simulink model "IEEE9_case"  (R2024b)
settings: Solver=FixedStepAuto  StartTime=0  StopTime=5  FixedStep=1e-7  RelTol=1e-3
values from neighbouring files (symbols this model uses):
  SG_D_1_D = 0.01056    [IEEE9_case_parameters.m]    (also in case1_parameters.m; case2_parameters.m; case3_parameters.m; case4_parameters.m)
  SG_D_1_EnableSaturation = 0    [IEEE9_case_parameters.m]    (also in case1_parameters.m; case2_parameters.m; case3_parameters.m; case4_parameters.m)
  SG_D_1_f0 = 60    [IEEE9_case_parameters.m]    (also in case1_parameters.m; case2_parameters.m; case3_parameters.m; case4_parameters.m)
  SG_D_1_H = 7.5    [IEEE9_case_parameters.m]    (also in case1_parameters.m; case2_parameters.m; case3_parameters.m; case4_parameters.m)
  SG_D_1_K_A = 20    [IEEE9_case_parameters.m]    (also in case1_parameters.m; case2_parameters.m; case3_parameters.m; case4_parameters.m)
  SG_D_1_K_E = 1.000000e+1    (= 10)    [IEEE9_case_parameters.m]    (also in case1_parameters.m; case2_parameters.m; case3_parameters.m; case4_parameters.m)
  SG_D_1_K_F = 2.363    [IEEE9_case_parameters.m]    (also in case1_parameters.m; case2_parameters.m; case3_parameters.m; case4_parameters.m)
  SG_D_1_K_s = 0.5    [IEEE9_case_parameters.m]    (also in case1_parameters.m = 5; case2_parameters.m = 5; case3_parameters.m = 5; case4_parameters.m = 5)
  SG_D_1_R_a = 0.001088    [IEEE9_case_parameters.m]    (also in case1_parameters.m; case2_parameters.m; case3_parameters.m; case4_parameters.m)
  SG_D_1_S_A = 1    [IEEE9_case_parameters.m]    (also in case1_parameters.m; case2_parameters.m; case3_parameters.m; case4_parameters.m)
  SG_D_1_S_B = 0.103    [IEEE9_case_parameters.m]    (also in case1_parameters.m; case2_parameters.m; case3_parameters.m; case4_parameters.m)
  SG_D_1_S_N = 10.659857    [IEEE9_case_parameters.m]    (also in case1_parameters.m; case2_parameters.m; case3_parameters.m; case4_parameters.m)
  SG_D_1_SpeedPara = 200    [IEEE9_case_parameters.m]    (also in case1_parameters.m; case2_parameters.m; case3_parameters.m; case4_parameters.m)
  SG_D_1_T_0 = 0.720173    [IEEE9_case_parameters.m]    (also in case1_parameters.m = 0.755522; case2_parameters.m = 0.808931; case3_parameters.m = 0.869402; case4_parameters.m = 0.729316)
  SG_D_1_T_1 = 0.3    [IEEE9_case_parameters.m]    (also in case1_parameters.m; case2_parameters.m; case3_parameters.m; case4_parameters.m)
  SG_D_1_T_2 = 0.05    [IEEE9_case_parameters.m]    (also in case1_parameters.m; case2_parameters.m; case3_parameters.m; case4_parameters.m)
  SG_D_1_T_3 = 0.02    [IEEE9_case_parameters.m]    (also in case1_parameters.m; case2_parameters.m; case3_parameters.m; case4_parameters.m)
  SG_D_1_T_4 = 0.005    [IEEE9_case_parameters.m]    (also in case1_parameters.m; case2_parameters.m; case3_parameters.m; case4_parameters.m)
  SG_D_1_T_A = 0.02    [IEEE9_case_parameters.m]    (also in case1_parameters.m; case2_parameters.m; case3_parameters.m; case4_parameters.m)
  SG_D_1_T_dd = 8.000000e+0    (= 8)    [IEEE9_case_parameters.m]    (also in case1_parameters.m; case2_parameters.m; case3_parameters.m; case4_parameters.m)
  SG_D_1_T_ddd = 0.04    [IEEE9_case_parameters.m]    (also in case1_parameters.m; case2_parameters.m; case3_parameters.m; case4_parameters.m)
  SG_D_1_T_E = 0.314    [IEEE9_case_parameters.m]    (also in case1_parameters.m; case2_parameters.m; case3_parameters.m; case4_parameters.m)
  SG_D_1_T_F = 0.35    [IEEE9_case_parameters.m]    (also in case1_parameters.m; case2_parameters.m; case3_parameters.m; case4_parameters.m)
  SG_D_1_T_qd = 0.8    [IEEE9_case_parameters.m]    (also in case1_parameters.m; case2_parameters.m; case3_parameters.m; case4_parameters.m)
  SG_D_1_T_qdd = 0.02    [IEEE9_case_parameters.m]    (also in case1_parameters.m; case2_parameters.m; case3_parameters.m; case4_parameters.m)
  SG_D_1_T_speed = 0.1    [IEEE9_case_parameters.m]    (also in case1_parameters.m = 200; case2_parameters.m = 200; case3_parameters.m = 200; case4_parameters.m = 200)
  SG_D_1_T_w = 0.5    [IEEE9_case_parameters.m]    (also in case1_parameters.m; case2_parameters.m; case3_parameters.m; case4_parameters.m)
  SG_D_1_V_ref = 1.990276    [IEEE9_case_parameters.m]    (also in case1_parameters.m = 2.042296; case2_parameters.m = 2.051388; case3_parameters.m = 2.089584; case4_parameters.m = 2.01845)
  SG_D_1_w_ref = 376.991118    [IEEE9_case_parameters.m]    (also in case1_parameters.m; case2_parameters.m; case3_parameters.m; case4_parameters.m)
  SG_D_1_wb = 6.000000e+1    (= 60)    [IEEE9_case_parameters.m]    (also in case1_parameters.m; case2_parameters.m; case3_parameters.m; case4_parameters.m)
  SG_D_1_x_d = 1.9    [IEEE9_case_parameters.m]    (also in case1_parameters.m; case2_parameters.m; case3_parameters.m; case4_parameters.m)
  SG_D_1_x_dd = 0.302    [IEEE9_case_parameters.m]    (also in case1_parameters.m; case2_parameters.m; case3_parameters.m; case4_parameters.m)
  SG_D_1_x_ddd = 0.204    [IEEE9_case_parameters.m]    (also in case1_parameters.m; case2_parameters.m; case3_parameters.m; case4_parameters.m)
  SG_D_1_x_l = 0.05    [IEEE9_case_parameters.m]    (also in case1_parameters.m; case2_parameters.m; case3_parameters.m; case4_parameters.m)
  SG_D_1_x_q = 1.3    [IEEE9_case_parameters.m]    (also in case1_parameters.m; case2_parameters.m; case3_parameters.m; case4_parameters.m)
  SG_D_1_x_qd = 0.5    [IEEE9_case_parameters.m]    (also in case1_parameters.m; case2_parameters.m; case3_parameters.m; case4_parameters.m)
  SG_D_1_x_qdd = 0.3    [IEEE9_case_parameters.m]    (also in case1_parameters.m; case2_parameters.m; case3_parameters.m; case4_parameters.m)
  SG_D_2_D = 0.02    [IEEE9_case_parameters.m]    (also in case1_parameters.m; case2_parameters.m; case3_parameters.m; case4_parameters.m)
  SG_D_2_EnableSaturation = 0    [IEEE9_case_parameters.m]    (also in case1_parameters.m; case2_parameters.m; case3_parameters.m; case4_parameters.m)
  SG_D_2_f0 = 60    [IEEE9_case_parameters.m]    (also in case1_parameters.m; case2_parameters.m; case3_parameters.m; case4_parameters.m)
  SG_D_2_H = 8.000000e+0    (= 8)    [IEEE9_case_parameters.m]    (also in case1_parameters.m; case2_parameters.m; case3_parameters.m; case4_parameters.m)
  SG_D_2_K_A = 20    [IEEE9_case_parameters.m]    (also in case1_parameters.m; case2_parameters.m; case3_parameters.m; case4_parameters.m)
  SG_D_2_K_E = 1.000000e+1    (= 10)    [IEEE9_case_parameters.m]    (also in case1_parameters.m; case2_parameters.m; case3_parameters.m; case4_parameters.m)
  SG_D_2_K_F = 2.363    [IEEE9_case_parameters.m]    (also in case1_parameters.m; case2_parameters.m; case3_parameters.m; case4_parameters.m)
  SG_D_2_K_s = 0.5    [IEEE9_case_parameters.m]    (also in case1_parameters.m = 4; case2_parameters.m = 4; case3_parameters.m = 4; case4_parameters.m = 4)
  SG_D_2_R_a = 0.001088    [IEEE9_case_parameters.m]    (also in case1_parameters.m; case2_parameters.m; case3_parameters.m; case4_parameters.m)
  SG_D_2_S_A = 1    [IEEE9_case_parameters.m]    (also in case1_parameters.m; case2_parameters.m; case3_parameters.m; case4_parameters.m)
  SG_D_2_S_B = 0.103    [IEEE9_case_parameters.m]    (also in case1_parameters.m; case2_parameters.m; case3_parameters.m; case4_parameters.m)
  SG_D_2_S_N = 10.659857    [IEEE9_case_parameters.m]    (also in case1_parameters.m; case2_parameters.m; case3_parameters.m; case4_parameters.m)
  SG_D_2_SpeedPara = 200    [IEEE9_case_parameters.m]    (also in case1_parameters.m; case2_parameters.m; case3_parameters.m; case4_parameters.m)
  SG_D_2_T_0 = 1.632913    [IEEE9_case_parameters.m]    (also in case1_parameters.m = 1.632925; case2_parameters.m = 1.632915; case3_parameters.m = 1.632914; case4_parameters.m = 1.632927)
  SG_D_2_T_1 = 0.2    [IEEE9_case_parameters.m]    (also in case1_parameters.m; case2_parameters.m; case3_parameters.m; case4_parameters.m)
  SG_D_2_T_2 = 0.05    [IEEE9_case_parameters.m]    (also in case1_parameters.m; case2_parameters.m; case3_parameters.m; case4_parameters.m)
  SG_D_2_T_3 = 0.02    [IEEE9_case_parameters.m]    (also in case1_parameters.m; case2_parameters.m; case3_parameters.m; case4_parameters.m)
  SG_D_2_T_4 = 0.005    [IEEE9_case_parameters.m]    (also in case1_parameters.m; case2_parameters.m; case3_parameters.m; case4_parameters.m)
  SG_D_2_T_A = 0.02    [IEEE9_case_parameters.m]    (also in case1_parameters.m; case2_parameters.m; case3_parameters.m; case4_parameters.m)
  SG_D_2_T_dd = 7.9    [IEEE9_case_parameters.m]    (also in case1_parameters.m; case2_parameters.m; case3_parameters.m; case4_parameters.m)
  SG_D_2_T_ddd = 0.04    [IEEE9_case_parameters.m]    (also in case1_parameters.m; case2_parameters.m; case3_parameters.m; case4_parameters.m)
  SG_D_2_T_E = 0.314    [IEEE9_case_parameters.m]    (also in case1_parameters.m; case2_parameters.m; case3_parameters.m; case4_parameters.m)
  SG_D_2_T_F = 0.35    [IEEE9_case_parameters.m]    (also in case1_parameters.m; case2_parameters.m; case3_parameters.m; case4_parameters.m)
  SG_D_2_T_qd = 0.8    [IEEE9_case_parameters.m]    (also in case1_parameters.m; case2_parameters.m; case3_parameters.m; case4_parameters.m)
  SG_D_2_T_qdd = 0.015    [IEEE9_case_parameters.m]    (also in case1_parameters.m; case2_parameters.m; case3_parameters.m; case4_parameters.m)
  SG_D_2_T_speed = 0.1    [IEEE9_case_parameters.m]    (also in case1_parameters.m = 150; case2_parameters.m = 150; case3_parameters.m = 150; case4_parameters.m = 150)
  SG_D_2_T_w = 0.35    [IEEE9_case_parameters.m]    (also in case1_parameters.m; case2_parameters.m; case3_parameters.m; case4_parameters.m)
  SG_D_2_V_ref = 2.58547    [IEEE9_case_parameters.m]    (also in case1_parameters.m = 2.597896; case2_parameters.m = 2.587136; case3_parameters.m = 2.586042; case4_parameters.m = 2.599679)
  SG_D_2_w_ref = 376.991118    [IEEE9_case_parameters.m]    (also in case1_parameters.m; case2_parameters.m; case3_parameters.m; case4_parameters.m)
  SG_D_2_wb = 6.000000e+1    (= 60)    [IEEE9_case_parameters.m]    (also in case1_parameters.m; case2_parameters.m; case3_parameters.m; case4_parameters.m)
  SG_D_2_x_d = 1.8    [IEEE9_case_parameters.m]    (also in case1_parameters.m; case2_parameters.m; case3_parameters.m; case4_parameters.m)
  SG_D_2_x_dd = 0.302    [IEEE9_case_parameters.m]    (also in case1_parameters.m; case2_parameters.m; case3_parameters.m; case4_parameters.m)
  SG_D_2_x_ddd = 0.204    [IEEE9_case_parameters.m]    (also in case1_parameters.m; case2_parameters.m; case3_parameters.m; case4_parameters.m)
  SG_D_2_x_l = 0.05    [IEEE9_case_parameters.m]    (also in case1_parameters.m; case2_parameters.m; case3_parameters.m; case4_parameters.m)
  SG_D_2_x_q = 1.25    [IEEE9_case_parameters.m]    (also in case1_parameters.m; case2_parameters.m; case3_parameters.m; case4_parameters.m)
  SG_D_2_x_qd = 0.5    [IEEE9_case_parameters.m]    (also in case1_parameters.m; case2_parameters.m; case3_parameters.m; case4_parameters.m)
  SG_D_2_x_qdd = 0.3    [IEEE9_case_parameters.m]    (also in case1_parameters.m; case2_parameters.m; case3_parameters.m; case4_parameters.m)
  SG_D_3_D = 0.02    [IEEE9_case_parameters.m]    (also in case1_parameters.m; case2_parameters.m; case3_parameters.m; case4_parameters.m)
  SG_D_3_EnableSaturation = 0    [IEEE9_case_parameters.m]    (also in case1_parameters.m; case2_parameters.m; case3_parameters.m; case4_parameters.m)
  SG_D_3_f0 = 60    [IEEE9_case_parameters.m]    (also in case1_parameters.m; case2_parameters.m; case3_parameters.m; case4_parameters.m)
  SG_D_3_H = 7.7    [IEEE9_case_parameters.m]    (also in case1_parameters.m; case2_parameters.m; case3_parameters.m; case4_parameters.m)
  SG_D_3_K_A = 20    [IEEE9_case_parameters.m]    (also in case1_parameters.m; case2_parameters.m; case3_parameters.m; case4_parameters.m)
  SG_D_3_K_E = 1.000000e+1    (= 10)    [IEEE9_case_parameters.m]    (also in case1_parameters.m; case2_parameters.m; case3_parameters.m; case4_parameters.m)
  SG_D_3_K_F = 2.363    [IEEE9_case_parameters.m]    (also in case1_parameters.m; case2_parameters.m; case3_parameters.m; case4_parameters.m)
  SG_D_3_K_s = 0.2    [IEEE9_case_parameters.m]    (also in case1_parameters.m = 2; case2_parameters.m = 2; case3_parameters.m = 2; case4_parameters.m = 2)
  SG_D_3_R_a = 0.001088    [IEEE9_case_parameters.m]    (also in case1_parameters.m; case2_parameters.m; case3_parameters.m; case4_parameters.m)
  SG_D_3_S_A = 1    [IEEE9_case_parameters.m]    (also in case1_parameters.m; case2_parameters.m; case3_parameters.m; case4_parameters.m)
  SG_D_3_S_B = 0.103    [IEEE9_case_parameters.m]    (also in case1_parameters.m; case2_parameters.m; case3_parameters.m; case4_parameters.m)
  SG_D_3_S_N = 10.659857    [IEEE9_case_parameters.m]    (also in case1_parameters.m; case2_parameters.m; case3_parameters.m; case4_parameters.m)
  SG_D_3_SpeedPara = 200    [IEEE9_case_parameters.m]    (also in case1_parameters.m; case2_parameters.m; case3_parameters.m; case4_parameters.m)
  SG_D_3_T_0 = 0.850788    [IEEE9_case_parameters.m]    (also in case1_parameters.m = 0.850786; case2_parameters.m = 0.850787; case3_parameters.m; case4_parameters.m = 0.850786)
  SG_D_3_T_1 = 0.2    [IEEE9_case_parameters.m]    (also in case1_parameters.m; case2_parameters.m; case3_parameters.m; case4_parameters.m)
  SG_D_3_T_2 = 0.05    [IEEE9_case_parameters.m]    (also in case1_parameters.m; case2_parameters.m; case3_parameters.m; case4_parameters.m)
  SG_D_3_T_3 = 0.02    [IEEE9_case_parameters.m]    (also in case1_parameters.m; case2_parameters.m; case3_parameters.m; case4_parameters.m)
  SG_D_3_T_4 = 0.005    [IEEE9_case_parameters.m]    (also in case1_parameters.m; case2_parameters.m; case3_parameters.m; case4_parameters.m)
  SG_D_3_T_A = 0.02    [IEEE9_case_parameters.m]    (also in case1_parameters.m; case2_parameters.m; case3_parameters.m; case4_parameters.m)
  SG_D_3_T_dd = 8.1    [IEEE9_case_parameters.m]    (also in case1_parameters.m; case2_parameters.m; case3_parameters.m; case4_parameters.m)
  SG_D_3_T_ddd = 0.04    [IEEE9_case_parameters.m]    (also in case1_parameters.m; case2_parameters.m; case3_parameters.m; case4_parameters.m)
  SG_D_3_T_E = 0.314    [IEEE9_case_parameters.m]    (also in case1_parameters.m; case2_parameters.m; case3_parameters.m; case4_parameters.m)
  SG_D_3_T_F = 0.35    [IEEE9_case_parameters.m]    (also in case1_parameters.m; case2_parameters.m; case3_parameters.m; case4_parameters.m)
  SG_D_3_T_qd = 0.8    [IEEE9_case_parameters.m]    (also in case1_parameters.m; case2_parameters.m; case3_parameters.m; case4_parameters.m)
  SG_D_3_T_qdd = 0.015    [IEEE9_case_parameters.m]    (also in case1_parameters.m; case2_parameters.m; case3_parameters.m; case4_parameters.m)
  SG_D_3_T_speed = 0.1    [IEEE9_case_parameters.m]    (also in case1_parameters.m = 180; case2_parameters.m = 180; case3_parameters.m = 180; case4_parameters.m = 180)
  SG_D_3_T_w = 0.4    [IEEE9_case_parameters.m]    (also in case1_parameters.m; case2_parameters.m; case3_parameters.m; case4_parameters.m)
  SG_D_3_V_ref = 1.892727    [IEEE9_case_parameters.m]    (also in case1_parameters.m = 1.906439; case2_parameters.m = 1.895535; case3_parameters.m = 1.892105; case4_parameters.m = 1.906598)
  SG_D_3_w_ref = 376.991118    [IEEE9_case_parameters.m]    (also in case1_parameters.m; case2_parameters.m; case3_parameters.m; case4_parameters.m)
  SG_D_3_wb = 6.000000e+1    (= 60)    [IEEE9_case_parameters.m]    (also in case1_parameters.m; case2_parameters.m; case3_parameters.m; case4_parameters.m)
  SG_D_3_x_d = 1.85    [IEEE9_case_parameters.m]    (also in case1_parameters.m; case2_parameters.m; case3_parameters.m; case4_parameters.m)
  SG_D_3_x_dd = 0.302    [IEEE9_case_parameters.m]    (also in case1_parameters.m; case2_parameters.m; case3_parameters.m; case4_parameters.m)
  SG_D_3_x_ddd = 0.204    [IEEE9_case_parameters.m]    (also in case1_parameters.m; case2_parameters.m; case3_parameters.m; case4_parameters.m)
  SG_D_3_x_l = 0.05    [IEEE9_case_parameters.m]    (also in case1_parameters.m; case2_parameters.m; case3_parameters.m; case4_parameters.m)
  SG_D_3_x_q = 1.2    [IEEE9_case_parameters.m]    (also in case1_parameters.m; case2_parameters.m; case3_parameters.m; case4_parameters.m)
  SG_D_3_x_qd = 0.5    [IEEE9_case_parameters.m]    (also in case1_parameters.m; case2_parameters.m; case3_parameters.m; case4_parameters.m)
  SG_D_3_x_qdd = 0.3    [IEEE9_case_parameters.m]    (also in case1_parameters.m; case2_parameters.m; case3_parameters.m; case4_parameters.m)
(part 10 of 12)

== system IEEE9_case/SG_D_3/d_R_f_SG_D_3_block ==
  note: d_R_f_SG_D_3 in IEEE9_case
      | $-\frac{R_{f,\mathrm{SG},D,3}-\frac{E_{\mathrm{fd},\mathrm{SG},D,3}\,K_{F}}{T_{F}}}{T_{F}}$
      | Automatically generated on 2025-11-01 08:50:13 .
  State_E_fd_SG_D_3_ddbea : Inport
  State_R_f_SG_D_3_c9e06 : Inport  Port=2
  Constant_K_F_22646 : Constant  Value=K_F
  Constant_T_F_0a0d1 : Constant  Value=T_F
  Constant_T_F_8804f : Constant  Value=T_F
  Divide_a64c1 : Product  Inputs=*/
  Divide_bf12f : Product  Inputs=*/
  Product_f7b73 : Product
  Subtract_0003f : Sum  Inputs=+-
  Blockout_d_R_f_SG_D_3_4784a : Outport
  wires:
  State_E_fd_SG_D_3_ddbea/1 -> Product_f7b73/1
  Constant_T_F_8804f/1 -> Divide_bf12f/2
  Constant_K_F_22646/1 -> Product_f7b73/2
  Product_f7b73/1 -> Divide_bf12f/1
  Divide_bf12f/1 -> Subtract_0003f/1
  State_R_f_SG_D_3_c9e06/1 -> Subtract_0003f/2
  Subtract_0003f/1 -> Divide_a64c1/1
  Constant_T_F_0a0d1/1 -> Divide_a64c1/2
  Divide_a64c1/1 -> Blockout_d_R_f_SG_D_3_4784a/1

== system IEEE9_case/SG_D_3/d_T_m_SG_D_3_block ==
  note: d_T_m_SG_D_3 in IEEE9_case
      | $-\frac{T_{m,\mathrm{SG},D,3}-T_{0}+\frac{\mathrm{SpeedPara}\,\left(w_{\mathrm{SG},D,3}-w_{\mathrm{ref}}\right)}{2\,f_{0}\,\pi }}{T_{\mathrm{speed}}}$
      | Automatically generated on 2025-11-01 08:50:04 .
  State_w_SG_D_3_50cf4 : Inport
  State_T_m_SG_D_3_a1980 : Inport  Port=2
  Add_41ff0 : Sum
  Add_ea0f0 : Sum
  Constant_-1_92da2 : Constant  Value=-1
  Constant_2.0_2378e : Constant  Value=2.0
  Constant_SpeedPara_095da : Constant  Value=SpeedPara
  Constant_T_0_75c83 : Constant  Value=T_0
  Constant_T_speed_09506 : Constant  Value=T_speed
  Constant_f0_b89eb : Constant  Value=f0
  Constant_pi_24d1e : Constant  Value=pi
  Constant_w_ref_fa68f : Constant  Value=w_ref
  Divide_5e003 : Product  Inputs=*/
  Divide_e250a : Product  Inputs=*/
  Product_43f4e : Product
  Product_b2d5f : Product
  Product_c70c6 : Product
  Product_f87e7 : Product
  Subtract_c06a0 : Sum  Inputs=+-
  Blockout_d_T_m_SG_D_3_5f1a1 : Outport
  wires:
  Constant_SpeedPara_095da/1 -> Product_f87e7/1
  Constant_-1_92da2/1 -> Product_b2d5f/1
  Constant_w_ref_fa68f/1 -> Add_ea0f0/2
  State_w_SG_D_3_50cf4/1 -> Product_b2d5f/2
  Constant_2.0_2378e/1 -> Product_c70c6/1
  Product_b2d5f/1 -> Add_ea0f0/1
  Constant_pi_24d1e/1 -> Product_c70c6/2
  Add_ea0f0/1 -> Product_f87e7/2
  Product_c70c6/1 -> Product_43f4e/1
  Constant_f0_b89eb/1 -> Product_43f4e/2
  Product_f87e7/1 -> Divide_e250a/1
  Product_43f4e/1 -> Divide_e250a/2
  Divide_e250a/1 -> Add_41ff0/1
  Constant_T_0_75c83/1 -> Add_41ff0/2
  Add_41ff0/1 -> Subtract_c06a0/1
  State_T_m_SG_D_3_a1980/1 -> Subtract_c06a0/2
  Subtract_c06a0/1 -> Divide_5e003/1
  Constant_T_speed_09506/1 -> Divide_5e003/2
  Divide_5e003/1 -> Blockout_d_T_m_SG_D_3_5f1a1/1

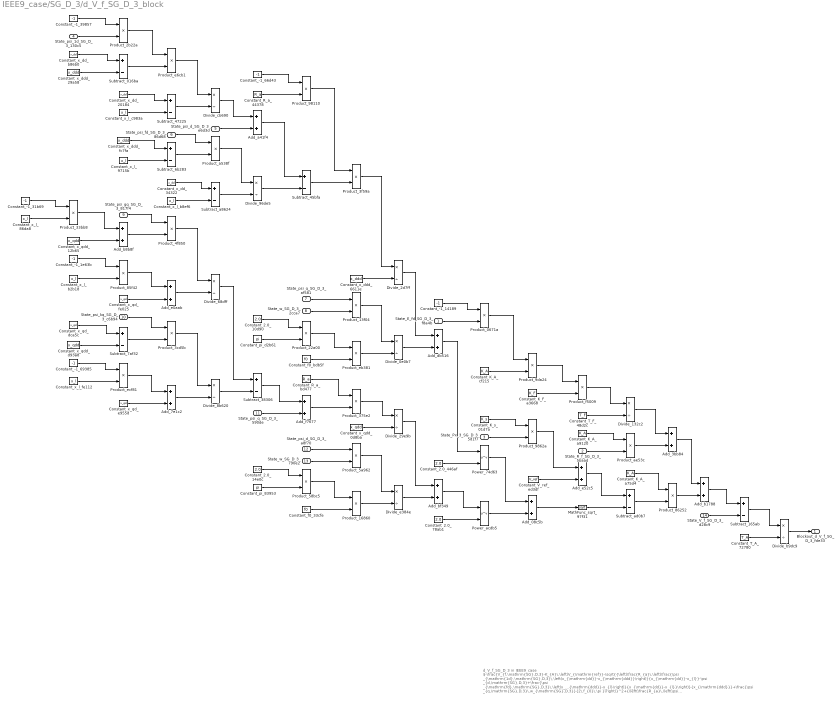
== system IEEE9_case/SG_D_3/d_V_f_SG_D_3_block ==
  note: d_V_f_SG_D_3 in IEEE9_case
      | $-\frac{V_{f,\mathrm{SG},D,3}-K_{A}\,\left(V_{\mathrm{ref}}-\sqrt{{\left(\frac{R_{a}\,\left(\frac{\psi _{\mathrm{1d},\mathrm{SG},D,3}\,\left(x_{\mathrm{dd}}-x_{\mathrm{ddd}}\right)}{x_{\mathrm{dd}}-x_{l}}-\psi _{d,\mathrm{SG},D,3}+\frac{\psi _{\mathrm{fd},\mathrm{SG},D,3}\,\left(x_{\mathrm{ddd}}-x_{l}\right)}{x_{\mathrm{dd}}-x_{l}}\right)}{x_{\mathrm{ddd}}}+\frac{\psi _{q,\mathrm{SG},D,3}\,w_{\mathrm{SG},D,3}}{2\,f_{0}\,\pi }\right)}^2+{\left(\frac{R_{a}\,\left(\psi _{q,\mathrm{SG},D,3}+\frac{\psi _{\mathrm{gq},\mathrm{SG},D,3}\,\left(x_{l}-x_{\mathrm{qdd}}\right)}{x_{l}-x_{\mathrm{qd}}}+\frac{\psi _{\mathrm{kq},\mathrm{SG},D,3}\,\left(x_{\mathrm{qd}}-x_{\mathrm{qdd}}\right)}{x_{l}-x_{\mathrm{qd}}}\right)}{x_{\mathrm{qdd}}}+\frac{\psi _{d,\mathrm{SG},D,3}\,w_{\mathrm{SG},D,3}}{2\,f_{0}\,\pi }\right)}^2}+K_{s}\,\mathrm{Px}_{3,\mathrm{SG},D,3}\right)-K_{A}\,R_{f,\mathrm{SG},D,3}+\frac{E_{\mathrm{fd},\mathrm{SG},D,3}\,K_{A}\,K_{F}}{T_{F}}}{T_{A}}$
      | Automatically generated on 2025-11-01 08:50:11 .
  State_E_fd_SG_D_3_f8a4b : Inport
  State_R_f_SG_D_3_5baad : Inport  Port=2
  State_Px_3_SG_D_3_5d1f7 : Inport  Port=3
  State_psi_1d_SG_D_3_130c5 : Inport  Port=4
  State_psi_d_SG_D_3_e6d3d : Inport  Port=5
  State_psi_fd_SG_D_3_86d68 : Inport  Port=6
  State_psi_q_SG_D_3_af581 : Inport  Port=7
  State_w_SG_D_3_2cca7 : Inport  Port=8
  State_psi_gq_SG_D_3_817f4 : Inport  Port=9
  State_psi_kq_SG_D_3_c6b94 : Inport  Port=10
  State_psi_q_SG_D_3_590de : Inport  Port=11
  State_psi_d_SG_D_3_a8f70 : Inport  Port=12
  State_w_SG_D_3_790e2 : Inport  Port=13
  State_V_f_SG_D_3_d28c9 : Inport  Port=14
  Add_08c5b : Sum
  Add_3bb84 : Sum
  Add_7e1c2 : Sum
  Add_a41f4 : Sum
  Add_b1788 : Sum
  Add_b8b8f : Sum
  Add_bf349 : Sum
  Add_db516 : Sum
  Add_e0aab : Sum
  Add_e52c5 : Sum
  Add_f7677 : Sum
  Constant_-1_14189 : Constant  Value=-1
  Constant_-1_1e63b : Constant  Value=-1
  Constant_-1_31b69 : Constant  Value=-1
  Constant_-1_39857 : Constant  Value=-1
  Constant_-1_66d43 : Constant  Value=-1
  Constant_-1_69385 : Constant  Value=-1
  Constant_2.0_10d90 : Constant  Value=2.0
  Constant_2.0_14e0c : Constant  Value=2.0
  Constant_2.0_446af : Constant  Value=2.0
  Constant_2.0_78ab1 : Constant  Value=2.0
  Constant_K_A_a75d4 : Constant  Value=K_A
  Constant_K_A_a9120 : Constant  Value=K_A
  Constant_K_A_cf215 : Constant  Value=K_A
  Constant_K_F_a3668 : Constant  Value=K_F
  Constant_K_s_01d7a : Constant  Value=K_s
  Constant_R_a_44378 : Constant  Value=R_a
  Constant_R_a_bd477 : Constant  Value=R_a
  Constant_T_A_72780 : Constant  Value=T_A
  Constant_T_F_48d2c : Constant  Value=T_F
  Constant_V_ref_ed3df : Constant  Value=V_ref
  Constant_f0_33cfe : Constant  Value=f0
  Constant_f0_bdb5f : Constant  Value=f0
  Constant_pi_83953 : Constant  Value=pi
  Constant_pi_d2b61 : Constant  Value=pi
  Constant_x_dd_20184 : Constant  Value=x_dd
  Constant_x_dd_34322 : Constant  Value=x_dd
  Constant_x_dd_b86b0 : Constant  Value=x_dd
  Constant_x_ddd_29a58 : Constant  Value=x_ddd
  Constant_x_ddd_6611e : Constant  Value=x_ddd
  Constant_x_ddd_fc7fa : Constant  Value=x_ddd
  Constant_x_l_86da8 : Constant  Value=x_l
  Constant_x_l_9715b : Constant  Value=x_l
  Constant_x_l_b2b18 : Constant  Value=x_l
  Constant_x_l_b8ef6 : Constant  Value=x_l
  Constant_x_l_c983a : Constant  Value=x_l
  Constant_x_l_fe112 : Constant  Value=x_l
  Constant_x_qd_dca5c : Constant  Value=x_qd
  Constant_x_qd_e955d : Constant  Value=x_qd
  Constant_x_qd_fe025 : Constant  Value=x_qd
  Constant_x_qdd_0d8ba : Constant  Value=x_qdd
  Constant_x_qdd_12b65 : Constant  Value=x_qdd
  Constant_x_qdd_d93a8 : Constant  Value=x_qdd
  Divide_0e0b7 : Product  Inputs=*/
  Divide_132c2 : Product  Inputs=*/
  Divide_29e9b : Product  Inputs=*/
  Divide_2d7ff : Product  Inputs=*/
  Divide_68dff : Product  Inputs=*/
  Divide_8b620 : Product  Inputs=*/
  Divide_96de5 : Product  Inputs=*/
  Divide_b9dc9 : Product  Inputs=*/
  Divide_cb690 : Product  Inputs=*/
  Divide_e384e : Product  Inputs=*/
  MathFunc_sqrt_97f31 : Sqrt
  Power_74d63 : Math  Operator=pow
  Power_acdb5 : Math  Operator=pow
  Product_0671a : Product
  Product_13f04 : Product
  Product_16860 : Product
  Product_22a00 : Product
  Product_2b22a : Product
  Product_33bb8 : Product
  Product_375e2 : Product
  Product_3cd5b : Product
  Product_3f59a : Product
  Product_4f850 : Product
  Product_58bc5 : Product
  Product_5a962 : Product
  Product_85f42 : Product
  Product_86252 : Product
  Product_98110 : Product
  Product_9862a : Product
  Product_9da24 : Product
  Product_a538f : Product
  Product_ae53c : Product
  Product_e6cb1 : Product
  Product_eb381 : Product
  Product_ecf81 : Product
  Product_f5009 : Product
  Subtract_016ba : Sum  Inputs=+-
  Subtract_165ab : Sum  Inputs=+-
  Subtract_38306 : Sum  Inputs=+-
  Subtract_45bfa : Sum  Inputs=+-
  Subtract_47225 : Sum  Inputs=+-
  Subtract_6b283 : Sum  Inputs=+-
  Subtract_7af32 : Sum  Inputs=+-
  Subtract_a8624 : Sum  Inputs=+-
  Subtract_ad0b7 : Sum  Inputs=+-
  Blockout_d_V_f_SG_D_3_fde33 : Outport
  wires:
  Constant_K_A_a9120/1 -> Product_ae53c/1
  Constant_-1_31b69/1 -> Product_33bb8/1
  Subtract_6b283/1 -> Product_a538f/2
  Constant_x_l_86da8/1 -> Product_33bb8/2
  Divide_e384e/1 -> Add_bf349/2
  Constant_-1_39857/1 -> Product_2b22a/1
  State_psi_1d_SG_D_3_130c5/1 -> Product_2b22a/2
  Constant_x_dd_b86b0/1 -> Subtract_016ba/1
  Divide_96de5/1 -> Subtract_45bfa/2
  Product_33bb8/1 -> Add_b8b8f/1
  Constant_x_qdd_12b65/1 -> Add_b8b8f/2
  Constant_x_ddd_29a58/1 -> Subtract_016ba/2
  Constant_2.0_78ab1/1 -> Power_acdb5/2
  Constant_-1_1e63b/1 -> Product_85f42/1
  Divide_68dff/1 -> Subtract_38306/1
  Subtract_47225/1 -> Divide_cb690/2
  Constant_x_l_b2b18/1 -> Product_85f42/2
  Constant_x_qd_dca5c/1 -> Subtract_7af32/1
  State_w_SG_D_3_2cca7/1 -> Product_13f04/2
  Constant_x_qdd_d93a8/1 -> Subtract_7af32/2
  Constant_2.0_10d90/1 -> Product_22a00/1
  Constant_-1_69385/1 -> Product_ecf81/1
  Constant_pi_d2b61/1 -> Product_22a00/2
  Add_a41f4/1 -> Subtract_45bfa/1
  Constant_x_l_fe112/1 -> Product_ecf81/2
  Product_2b22a/1 -> Product_e6cb1/1
  Subtract_016ba/1 -> Product_e6cb1/2
  Constant_2.0_14e0c/1 -> Product_58bc5/1
  Constant_x_dd_20184/1 -> Subtract_47225/1
  Constant_pi_83953/1 -> Product_58bc5/2
  Constant_x_l_c983a/1 -> Subtract_47225/2
  Constant_x_ddd_fc7fa/1 -> Subtract_6b283/1
  Constant_x_l_9715b/1 -> Subtract_6b283/2
  State_psi_gq_SG_D_3_817f4/1 -> Product_4f850/1
  Constant_x_l_b8ef6/1 -> Subtract_a8624/2
  Add_b8b8f/1 -> Product_4f850/2
  Product_85f42/1 -> Add_e0aab/1
  Product_4f850/1 -> Divide_68dff/1
  Constant_x_qd_fe025/1 -> Add_e0aab/2
  State_psi_kq_SG_D_3_c6b94/1 -> Product_3cd5b/1
  State_psi_q_SG_D_3_af581/1 -> Product_13f04/1
  Add_db516/1 -> Power_74d63/1
  Subtract_7af32/1 -> Product_3cd5b/2
  Constant_f0_bdb5f/1 -> Product_eb381/2
  Product_22a00/1 -> Product_eb381/1
  Constant_x_qd_e955d/1 -> Add_7e1c2/2
  Product_ecf81/1 -> Add_7e1c2/1
  Product_e6cb1/1 -> Divide_cb690/1
  State_psi_fd_SG_D_3_86d68/1 -> Product_a538f/1
  Constant_x_dd_34322/1 -> Subtract_a8624/1
  Add_e0aab/1 -> Divide_68dff/2
  Add_08c5b/1 -> MathFunc_sqrt_97f31/1
  Product_3cd5b/1 -> Divide_8b620/1
  Add_7e1c2/1 -> Divide_8b620/2
  Product_98110/1 -> Product_3f59a/1
  Divide_cb690/1 -> Add_a41f4/1
  Add_e52c5/1 -> Subtract_ad0b7/1
  State_psi_d_SG_D_3_e6d3d/1 -> Add_a41f4/2
  Product_a538f/1 -> Divide_96de5/1
  Subtract_a8624/1 -> Divide_96de5/2
  MathFunc_sqrt_97f31/1 -> Subtract_ad0b7/2
  Divide_8b620/1 -> Subtract_38306/2
  Constant_-1_66d43/1 -> Product_98110/1
  Constant_R_a_44378/1 -> Product_98110/2
  Subtract_38306/1 -> Add_f7677/1
  State_psi_q_SG_D_3_590de/1 -> Add_f7677/2
  Subtract_45bfa/1 -> Product_3f59a/2
  Constant_R_a_bd477/1 -> Product_375e2/1
  Add_f7677/1 -> Product_375e2/2
  State_psi_d_SG_D_3_a8f70/1 -> Product_5a962/1
  State_w_SG_D_3_790e2/1 -> Product_5a962/2
  Product_58bc5/1 -> Product_16860/1
  Constant_f0_33cfe/1 -> Product_16860/2
  Product_3f59a/1 -> Divide_2d7ff/1
  Constant_x_ddd_6611e/1 -> Divide_2d7ff/2
  Product_13f04/1 -> Divide_0e0b7/1
  Product_eb381/1 -> Divide_0e0b7/2
  Product_375e2/1 -> Divide_29e9b/1
  Constant_x_qdd_0d8ba/1 -> Divide_29e9b/2
  Product_5a962/1 -> Divide_e384e/1
  Product_16860/1 -> Divide_e384e/2
  Divide_2d7ff/1 -> Add_db516/1
  Divide_0e0b7/1 -> Add_db516/2
  Divide_29e9b/1 -> Add_bf349/1
  Constant_-1_14189/1 -> Product_0671a/1
  State_E_fd_SG_D_3_f8a4b/1 -> Product_0671a/2
  Constant_2.0_446af/1 -> Power_74d63/2
  Add_bf349/1 -> Power_acdb5/1
  Product_0671a/1 -> Product_9da24/1
  Constant_K_A_cf215/1 -> Product_9da24/2
  Constant_K_s_01d7a/1 -> Product_9862a/1
  State_Px_3_SG_D_3_5d1f7/1 -> Product_9862a/2
  Power_74d63/1 -> Add_08c5b/1
  Power_acdb5/1 -> Add_08c5b/2
  Product_9da24/1 -> Product_f5009/1
  Constant_K_F_a3668/1 -> Product_f5009/2
  Product_9862a/1 -> Add_e52c5/1
  Constant_V_ref_ed3df/1 -> Add_e52c5/2
  Product_f5009/1 -> Divide_132c2/1
  Constant_T_F_48d2c/1 -> Divide_132c2/2
  Add_b1788/1 -> Subtract_165ab/1
  State_R_f_SG_D_3_5baad/1 -> Product_ae53c/2
  Divide_132c2/1 -> Add_3bb84/1
  Product_ae53c/1 -> Add_3bb84/2
  Constant_K_A_a75d4/1 -> Product_86252/1
  Subtract_ad0b7/1 -> Product_86252/2
  Add_3bb84/1 -> Add_b1788/1
  Product_86252/1 -> Add_b1788/2
  State_V_f_SG_D_3_d28c9/1 -> Subtract_165ab/2
  Subtract_165ab/1 -> Divide_b9dc9/1
  Constant_T_A_72780/1 -> Divide_b9dc9/2
  Divide_b9dc9/1 -> Blockout_d_V_f_SG_D_3_fde33/1

== system IEEE9_case/SG_D_3/d_psi_1d_SG_D_3_block ==
  note: d_psi_1d_SG_D_3 in IEEE9_case
      | $-\frac{\psi _{\mathrm{1d},\mathrm{SG},D,3}-\psi _{\mathrm{fd},\mathrm{SG},D,3}+\frac{\left(x_{\mathrm{dd}}-x_{l}\right)\,\left(\frac{\psi _{\mathrm{1d},\mathrm{SG},D,3}\,\left(x_{\mathrm{dd}}-x_{\mathrm{ddd}}\right)}{x_{\mathrm{dd}}-x_{l}}-\psi _{d,\mathrm{SG},D,3}+\frac{\psi _{\mathrm{fd},\mathrm{SG},D,3}\,\left(x_{\mathrm{ddd}}-x_{l}\right)}{x_{\mathrm{dd}}-x_{l}}\right)}{x_{\mathrm{ddd}}}}{T_{\mathrm{ddd}}}$
      | Automatically generated on 2025-11-01 08:49:48 .
  State_psi_1d_SG_D_3_dcaf3 : Inport
  State_psi_fd_SG_D_3_cacc3 : Inport  Port=2
  State_psi_1d_SG_D_3_98130 : Inport  Port=3
  State_psi_d_SG_D_3_fbd14 : Inport  Port=4
  State_psi_fd_SG_D_3_9f125 : Inport  Port=5
  Add_15da8 : Sum
  Add_83c0c : Sum
  Add_a7352 : Sum
  Constant_-1_18e36 : Constant  Value=-1
  Constant_-1_dc142 : Constant  Value=-1
  Constant_T_ddd_806da : Constant  Value=T_ddd
  Constant_x_dd_4b99c : Constant  Value=x_dd
  Constant_x_dd_76a92 : Constant  Value=x_dd
  Constant_x_dd_af030 : Constant  Value=x_dd
  Constant_x_dd_f0d56 : Constant  Value=x_dd
  Constant_x_ddd_4ece0 : Constant  Value=x_ddd
  Constant_x_ddd_688f3 : Constant  Value=x_ddd
  Constant_x_ddd_b84f1 : Constant  Value=x_ddd
  Constant_x_l_8316f : Constant  Value=x_l
  Constant_x_l_95cb8 : Constant  Value=x_l
  Constant_x_l_b4d52 : Constant  Value=x_l
  Constant_x_l_eaaef : Constant  Value=x_l
  Divide_065c3 : Product  Inputs=*/
  Divide_14861 : Product  Inputs=*/
  Divide_3c16f : Product  Inputs=*/
  Divide_4ed99 : Product  Inputs=*/
  Product_14a64 : Product
  Product_74950 : Product
  Product_afc25 : Product
  Product_b95af : Product
  Product_d3848 : Product
  Subtract_0f08b : Sum  Inputs=+-
  Subtract_361bd : Sum  Inputs=+-
  Subtract_4fe76 : Sum  Inputs=+-
  Subtract_70533 : Sum  Inputs=+-
  Subtract_7fade : Sum  Inputs=+-
  Subtract_922fb : Sum  Inputs=+-
  Blockout_d_psi_1d_SG_D_3_549d8 : Outport
  wires:
  Divide_14861/1 -> Add_15da8/1
  Subtract_361bd/1 -> Product_afc25/2
  Constant_-1_dc142/1 -> Product_74950/1
  Constant_x_dd_f0d56/1 -> Subtract_4fe76/1
  State_psi_1d_SG_D_3_98130/1 -> Product_74950/2
  Product_74950/1 -> Product_afc25/1
  Constant_x_dd_76a92/1 -> Subtract_361bd/1
  Constant_x_ddd_688f3/1 -> Subtract_361bd/2
  Constant_x_l_95cb8/1 -> Subtract_4fe76/2
  Constant_x_ddd_b84f1/1 -> Subtract_70533/1
  Divide_3c16f/1 -> Blockout_d_psi_1d_SG_D_3_549d8/1
  Constant_x_l_b4d52/1 -> Subtract_70533/2
  Product_afc25/1 -> Divide_14861/1
  Subtract_4fe76/1 -> Divide_14861/2
  State_psi_fd_SG_D_3_9f125/1 -> Product_14a64/1
  Subtract_70533/1 -> Product_14a64/2
  Constant_x_dd_af030/1 -> Subtract_0f08b/1
  Constant_x_l_eaaef/1 -> Subtract_0f08b/2
  State_psi_d_SG_D_3_fbd14/1 -> Add_15da8/2
  Product_14a64/1 -> Divide_065c3/1
  Subtract_0f08b/1 -> Divide_065c3/2
  Constant_x_dd_4b99c/1 -> Subtract_922fb/1
  Constant_x_l_8316f/1 -> Subtract_922fb/2
  Add_15da8/1 -> Subtract_7fade/1
  Divide_065c3/1 -> Subtract_7fade/2
  Constant_-1_18e36/1 -> Product_d3848/1
  State_psi_1d_SG_D_3_dcaf3/1 -> Product_d3848/2
  State_psi_fd_SG_D_3_cacc3/1 -> Add_83c0c/2
  Subtract_922fb/1 -> Product_b95af/1
  Subtract_7fade/1 -> Product_b95af/2
  Product_d3848/1 -> Add_83c0c/1
  Product_b95af/1 -> Divide_4ed99/1
  Constant_x_ddd_4ece0/1 -> Divide_4ed99/2
  Add_83c0c/1 -> Add_a7352/1
  Divide_4ed99/1 -> Add_a7352/2
  Add_a7352/1 -> Divide_3c16f/1
  Constant_T_ddd_806da/1 -> Divide_3c16f/2

== system IEEE9_case/SG_D_3/d_psi_d_SG_D_3_block ==
  note: d_psi_d_SG_D_3 in IEEE9_case
      | $2\,\pi \,f_{0}\,\left(v_{d,\mathrm{SG},D,3}\,\sin\left(\theta _{\mathrm{SG},D,3}\right)-v_{q,\mathrm{SG},D,3}\,\cos\left(\theta _{\mathrm{SG},D,3}\right)+\frac{R_{a}\,\left(\frac{\psi _{\mathrm{1d},\mathrm{SG},D,3}\,\left(x_{\mathrm{dd}}-x_{\mathrm{ddd}}\right)}{x_{\mathrm{dd}}-x_{l}}-\psi _{d,\mathrm{SG},D,3}+\frac{\psi _{\mathrm{fd},\mathrm{SG},D,3}\,\left(x_{\mathrm{ddd}}-x_{l}\right)}{x_{\mathrm{dd}}-x_{l}}\right)}{x_{\mathrm{ddd}}}+\frac{\psi _{q,\mathrm{SG},D,3}\,w_{\mathrm{SG},D,3}}{2\,f_{0}\,\pi }\right)$
      | Automatically generated on 2025-11-01 08:49:39 .
  State_psi_1d_SG_D_3_ec6d7 : Inport
  State_psi_d_SG_D_3_cd386 : Inport  Port=2
  State_psi_fd_SG_D_3_f7fa4 : Inport  Port=3
  Input_v_d_SG_D_3_c1082 : Inport  Port=4
  State_theta_SG_D_3_79acd : Inport  Port=5
  Input_v_q_SG_D_3_d2650 : Inport  Port=6
  State_theta_SG_D_3_d0ec2 : Inport  Port=7
  State_psi_q_SG_D_3_63db3 : Inport  Port=8
  State_w_SG_D_3_c8b72 : Inport  Port=9
  Add_7d94c : Sum
  Add_c23eb : Sum
  Constant_-1_b66cc : Constant  Value=-1
  Constant_-2.0_d9ac7 : Constant  Value=-2.0
  Constant_2.0_7e810 : Constant  Value=2.0
  Constant_R_a_5fc7e : Constant  Value=R_a
  Constant_f0_5bc15 : Constant  Value=f0
  Constant_f0_8268e : Constant  Value=f0
  Constant_pi_02ee2 : Constant  Value=pi
  Constant_pi_d37fe : Constant  Value=pi
  Constant_x_dd_0ce51 : Constant  Value=x_dd
  Constant_x_dd_5686e : Constant  Value=x_dd
  Constant_x_dd_6e989 : Constant  Value=x_dd
  Constant_x_ddd_32dbf : Constant  Value=x_ddd
  Constant_x_ddd_6e6b5 : Constant  Value=x_ddd
  Constant_x_ddd_9b171 : Constant  Value=x_ddd
  Constant_x_l_1451d : Constant  Value=x_l
  Constant_x_l_c1c50 : Constant  Value=x_l
  Constant_x_l_e75f6 : Constant  Value=x_l
  Divide_30391 : Product  Inputs=*/
  Divide_bb8a0 : Product  Inputs=*/
  Divide_bebb2 : Product  Inputs=*/
  Divide_e0f9d : Product  Inputs=*/
  MathFunc_cos_fdc9f : Trigonometry  Operator=cos
  MathFunc_sin_20479 : Trigonometry
  Product_0c9b7 : Product
  Product_1403c : Product
  Product_1465a : Product
  Product_31711 : Product
  Product_485fb : Product
  Product_7d538 : Product
  Product_7f1be : Product
  Product_87be9 : Product
  Product_8f97a : Product
  Product_a0011 : Product
  Product_f637c : Product
  Product_f7ca5 : Product
  Subtract_09f13 : Sum  Inputs=+-
  Subtract_21e04 : Sum  Inputs=+-
  Subtract_30b02 : Sum  Inputs=+-
  Subtract_a3228 : Sum  Inputs=+-
  Subtract_b7ec2 : Sum  Inputs=+-
  Subtract_fc50a : Sum  Inputs=+-
  Subtract_ffcf7 : Sum  Inputs=+-
  Blockout_d_psi_d_SG_D_3_12622 : Outport
  wires:
  Constant_-1_b66cc/1 -> Product_0c9b7/1
  Constant_2.0_7e810/1 -> Product_87be9/1
  Constant_x_dd_5686e/1 -> Subtract_30b02/1
  State_psi_1d_SG_D_3_ec6d7/1 -> Product_0c9b7/2
  Constant_x_dd_0ce51/1 -> Subtract_b7ec2/1
  Constant_pi_02ee2/1 -> Product_87be9/2
  Constant_x_ddd_9b171/1 -> Subtract_30b02/2
  Product_0c9b7/1 -> Product_31711/1
  Product_87be9/1 -> Product_f7ca5/1
  Subtract_30b02/1 -> Product_31711/2
  Constant_-2.0_d9ac7/1 -> Product_a0011/1
  Constant_x_l_c1c50/1 -> Subtract_b7ec2/2
  Constant_x_ddd_32dbf/1 -> Subtract_a3228/1
  Constant_pi_d37fe/1 -> Product_a0011/2
  Constant_x_l_1451d/1 -> Subtract_a3228/2
  Product_7d538/1 -> Divide_30391/1
  Product_31711/1 -> Divide_bebb2/1
  Subtract_b7ec2/1 -> Divide_bebb2/2
  State_psi_fd_SG_D_3_f7fa4/1 -> Product_485fb/1
  Subtract_a3228/1 -> Product_485fb/2
  Constant_x_dd_6e989/1 -> Subtract_21e04/1
  Constant_x_l_e75f6/1 -> Subtract_21e04/2
  Divide_30391/1 -> Subtract_09f13/2
  Divide_bebb2/1 -> Add_7d94c/1
  Subtract_fc50a/1 -> Product_7f1be/2
  State_psi_d_SG_D_3_cd386/1 -> Add_7d94c/2
  Product_485fb/1 -> Divide_bb8a0/1
  Subtract_21e04/1 -> Divide_bb8a0/2
  Add_7d94c/1 -> Subtract_fc50a/1
  Divide_bb8a0/1 -> Subtract_fc50a/2
  Product_f637c/1 -> Add_c23eb/2
  Constant_R_a_5fc7e/1 -> Product_7f1be/1
  Product_1465a/1 -> Product_1403c/1
  State_theta_SG_D_3_79acd/1 -> MathFunc_sin_20479/1
  Product_7f1be/1 -> Divide_e0f9d/1
  Constant_x_ddd_6e6b5/1 -> Divide_e0f9d/2
  Input_v_d_SG_D_3_c1082/1 -> Product_8f97a/1
  State_w_SG_D_3_c8b72/1 -> Product_7d538/2
  MathFunc_sin_20479/1 -> Product_8f97a/2
  State_theta_SG_D_3_d0ec2/1 -> MathFunc_cos_fdc9f/1
  MathFunc_cos_fdc9f/1 -> Product_f637c/2
  Divide_e0f9d/1 -> Subtract_ffcf7/1
  Product_8f97a/1 -> Subtract_ffcf7/2
  Input_v_q_SG_D_3_d2650/1 -> Product_f637c/1
  State_psi_q_SG_D_3_63db3/1 -> Product_7d538/1
  Constant_f0_8268e/1 -> Product_f7ca5/2
  Subtract_ffcf7/1 -> Add_c23eb/1
  Product_f7ca5/1 -> Divide_30391/2
  Product_a0011/1 -> Product_1465a/1
  Constant_f0_5bc15/1 -> Product_1465a/2
  Add_c23eb/1 -> Subtract_09f13/1
  Subtract_09f13/1 -> Product_1403c/2
  Product_1403c/1 -> Blockout_d_psi_d_SG_D_3_12622/1

== system IEEE9_case/SG_D_3/d_psi_fd_SG_D_3_block ==
  note: d_psi_fd_SG_D_3 in IEEE9_case
      | $-\frac{\psi _{\mathrm{fd},\mathrm{SG},D,3}-E_{\mathrm{fd},\mathrm{SG},D,3}+\left(x_{d}-x_{\mathrm{dd}}\right)\,\left(\frac{\frac{\psi _{\mathrm{1d},\mathrm{SG},D,3}\,\left(x_{\mathrm{dd}}-x_{\mathrm{ddd}}\right)}{x_{\mathrm{dd}}-x_{l}}-\psi _{d,\mathrm{SG},D,3}+\frac{\psi _{\mathrm{fd},\mathrm{SG},D,3}\,\left(x_{\mathrm{ddd}}-x_{l}\right)}{x_{\mathrm{dd}}-x_{l}}}{x_{\mathrm{ddd}}}-\frac{\left(x_{\mathrm{dd}}-x_{\mathrm{ddd}}\right)\,\left(\psi _{\mathrm{1d},\mathrm{SG},D,3}-\psi _{\mathrm{fd},\mathrm{SG},D,3}+\frac{\left(x_{\mathrm{dd}}-x_{l}\right)\,\left(\frac{\psi _{\mathrm{1d},\mathrm{SG},D,3}\,\left(x_{\mathrm{dd}}-x_{\mathrm{ddd}}\right)}{x_{\mathrm{dd}}-x_{l}}-\psi _{d,\mathrm{SG},D,3}+\frac{\psi _{\mathrm{fd},\mathrm{SG},D,3}\,\left(x_{\mathrm{ddd}}-x_{l}\right)}{x_{\mathrm{dd}}-x_{l}}\right)}{x_{\mathrm{ddd}}}\right)}{{\left(x_{\mathrm{dd}}-x_{l}\right)}^2}\right)}{T_{\mathrm{dd}}}$
      | Automatically generated on 2025-11-01 08:49:46 .
  State_E_fd_SG_D_3_68bde : Inport
  State_psi_fd_SG_D_3_dfb80 : Inport  Port=2
  State_psi_1d_SG_D_3_bd0db : Inport  Port=3
  State_psi_fd_SG_D_3_019c6 : Inport  Port=4
  State_psi_1d_SG_D_3_eed35 : Inport  Port=5
  State_psi_d_SG_D_3_bb63b : Inport  Port=6
  State_psi_fd_SG_D_3_c7d54 : Inport  Port=7
  State_psi_1d_SG_D_3_a1855 : Inport  Port=8
  State_psi_d_SG_D_3_9ca4c : Inport  Port=9
  State_psi_fd_SG_D_3_c8342 : Inport  Port=10
  Add_66feb : Sum
  Add_d4d18 : Sum
  Constant_-1_07103 : Constant  Value=-1
  Constant_-1_74707 : Constant  Value=-1
  Constant_-1_d240c : Constant  Value=-1
  Constant_2.0_4357e : Constant  Value=2.0
  Constant_T_dd_28a4a : Constant  Value=T_dd
  Constant_x_d_05f42 : Constant  Value=x_d
  Constant_x_dd_01978 : Constant  Value=x_dd
  Constant_x_dd_01ff1 : Constant  Value=x_dd
  Constant_x_dd_0db39 : Constant  Value=x_dd
  Constant_x_dd_17aff : Constant  Value=x_dd
  Constant_x_dd_21fef : Constant  Value=x_dd
  Constant_x_dd_587d6 : Constant  Value=x_dd
  Constant_x_dd_7dafa : Constant  Value=x_dd
  Constant_x_dd_8a7ab : Constant  Value=x_dd
  Constant_x_dd_bbea0 : Constant  Value=x_dd
  Constant_x_dd_fa49f : Constant  Value=x_dd
  Constant_x_ddd_22fc5 : Constant  Value=x_ddd
  Constant_x_ddd_329fc : Constant  Value=x_ddd
  Constant_x_ddd_4687a : Constant  Value=x_ddd
  Constant_x_ddd_5047a : Constant  Value=x_ddd
  Constant_x_ddd_53329 : Constant  Value=x_ddd
  Constant_x_ddd_7fc11 : Constant  Value=x_ddd
  Constant_x_ddd_93d40 : Constant  Value=x_ddd
  Constant_x_l_058d7 : Constant  Value=x_l
  Constant_x_l_14bd6 : Constant  Value=x_l
  Constant_x_l_1a133 : Constant  Value=x_l
  Constant_x_l_31fc2 : Constant  Value=x_l
  Constant_x_l_3582d : Constant  Value=x_l
  Constant_x_l_b9ee2 : Constant  Value=x_l
  Constant_x_l_fe475 : Constant  Value=x_l
  Constant_x_l_ff0d1 : Constant  Value=x_l
  Divide_60e18 : Product  Inputs=*/
  Divide_76588 : Product  Inputs=*/
  Divide_8510e : Product  Inputs=*/
  Divide_adb28 : Product  Inputs=*/
  Divide_c596a : Product  Inputs=*/
  Divide_e38e5 : Product  Inputs=*/
  Divide_e72f7 : Product  Inputs=*/
  Divide_fd089 : Product  Inputs=*/
  Power_dd6db : Math  Operator=pow
  Product_0f774 : Product
  Product_175fb : Product
  Product_272d2 : Product
  Product_2ee51 : Product
  Product_342c2 : Product
  Product_95daa : Product
  Product_bf137 : Product
  Product_ccd13 : Product
  Product_ee2bc : Product
  Product_efc4d : Product
  Subtract_0f54f : Sum  Inputs=+-
  Subtract_10d39 : Sum  Inputs=+-
  Subtract_1c09f : Sum  Inputs=+-
  Subtract_2a797 : Sum  Inputs=+-
  Subtract_331b2 : Sum  Inputs=+-
  Subtract_3d09a : Sum  Inputs=+-
  Subtract_4061c : Sum  Inputs=+-
  Subtract_40994 : Sum  Inputs=+-
  Subtract_4fde8 : Sum  Inputs=+-
  Subtract_51ab9 : Sum  Inputs=+-
  Subtract_5baa0 : Sum  Inputs=+-
  Subtract_68f18 : Sum  Inputs=+-
  Subtract_6df93 : Sum  Inputs=+-
  Subtract_91f4e : Sum  Inputs=+-
  Subtract_a651a : Sum  Inputs=+-
  Subtract_b4e06 : Sum  Inputs=+-
  Subtract_b9ff4 : Sum  Inputs=+-
  Subtract_c6879 : Sum  Inputs=+-
  Subtract_eb416 : Sum  Inputs=+-
  Blockout_d_psi_fd_SG_D_3_68982 : Outport
  wires:
  Product_ccd13/1 -> Divide_e72f7/1
  Constant_-1_d240c/1 -> Product_95daa/1
  Subtract_b9ff4/1 -> Product_ee2bc/2
  State_psi_1d_SG_D_3_eed35/1 -> Product_95daa/2
  Constant_x_l_1a133/1 -> Subtract_10d39/2
  Constant_x_dd_fa49f/1 -> Subtract_b9ff4/1
  Constant_x_ddd_53329/1 -> Subtract_b9ff4/2
  Product_95daa/1 -> Product_ee2bc/1
  Constant_x_dd_7dafa/1 -> Subtract_5baa0/1
  Constant_x_l_14bd6/1 -> Subtract_5baa0/2
  Constant_x_ddd_93d40/1 -> Subtract_0f54f/2
  Constant_x_ddd_4687a/1 -> Subtract_40994/1
  Constant_x_l_ff0d1/1 -> Subtract_40994/2
  Product_bf137/1 -> Product_0f774/1
  Product_ee2bc/1 -> Divide_e38e5/1
  Subtract_5baa0/1 -> Divide_e38e5/2
  State_psi_fd_SG_D_3_c7d54/1 -> Product_efc4d/1
  Constant_x_ddd_5047a/1 -> Subtract_10d39/1
  Subtract_40994/1 -> Product_efc4d/2
  Constant_x_dd_587d6/1 -> Subtract_51ab9/1
  Constant_-1_74707/1 -> Product_bf137/1
  Constant_x_l_31fc2/1 -> Subtract_51ab9/2
  Product_0f774/1 -> Divide_76588/1
  Divide_e38e5/1 -> Add_d4d18/1
  Product_272d2/1 -> Divide_60e18/1
  State_psi_d_SG_D_3_bb63b/1 -> Add_d4d18/2
  State_psi_fd_SG_D_3_c8342/1 -> Product_272d2/1
  Product_efc4d/1 -> Divide_adb28/1
  Constant_x_dd_8a7ab/1 -> Subtract_4fde8/1
  Subtract_51ab9/1 -> Divide_adb28/2
  Constant_x_l_058d7/1 -> Subtract_2a797/2
  Constant_x_dd_0db39/1 -> Subtract_c6879/1
  Subtract_91f4e/1 -> Product_175fb/2
  Constant_x_l_3582d/1 -> Subtract_c6879/2
  Divide_76588/1 -> Add_66feb/1
  Constant_x_ddd_329fc/1 -> Divide_e72f7/2
  Add_d4d18/1 -> Subtract_b4e06/1
  Divide_adb28/1 -> Subtract_b4e06/2
  State_psi_1d_SG_D_3_a1855/1 -> Product_bf137/2
  Constant_x_l_b9ee2/1 -> Subtract_4fde8/2
  Constant_x_dd_01978/1 -> Subtract_0f54f/1
  Subtract_c6879/1 -> Product_ccd13/1
  Add_66feb/1 -> Subtract_3d09a/1
  Subtract_b4e06/1 -> Product_ccd13/2
  Subtract_0f54f/1 -> Product_0f774/2
  Constant_x_dd_bbea0/1 -> Subtract_4061c/1
  Constant_x_l_fe475/1 -> Subtract_4061c/2
  Subtract_10d39/1 -> Product_272d2/2
  Constant_x_dd_01ff1/1 -> Subtract_91f4e/1
  Constant_x_ddd_7fc11/1 -> Subtract_91f4e/2
  Product_175fb/1 -> Product_2ee51/1
  State_psi_1d_SG_D_3_bd0db/1 -> Subtract_68f18/1
  Subtract_4061c/1 -> Divide_76588/2
  State_psi_fd_SG_D_3_019c6/1 -> Subtract_68f18/2
  Constant_-1_07103/1 -> Product_175fb/1
  Subtract_68f18/1 -> Subtract_a651a/1
  Divide_e72f7/1 -> Subtract_a651a/2
  Constant_x_dd_17aff/1 -> Subtract_2a797/1
  Divide_60e18/1 -> Subtract_3d09a/2
  State_psi_d_SG_D_3_9ca4c/1 -> Add_66feb/2
  Subtract_4fde8/1 -> Divide_60e18/2
  Subtract_a651a/1 -> Product_2ee51/2
  Subtract_2a797/1 -> Power_dd6db/1
  Constant_2.0_4357e/1 -> Power_dd6db/2
  Product_2ee51/1 -> Divide_fd089/1
  Subtract_331b2/1 -> Product_342c2/2
  Power_dd6db/1 -> Divide_fd089/2
  Subtract_3d09a/1 -> Divide_8510e/1
  Constant_x_ddd_22fc5/1 -> Divide_8510e/2
  Constant_x_d_05f42/1 -> Subtract_eb416/1
  Constant_x_dd_21fef/1 -> Subtract_eb416/2
  Divide_fd089/1 -> Subtract_331b2/1
  Divide_8510e/1 -> Subtract_331b2/2
  State_E_fd_SG_D_3_68bde/1 -> Subtract_1c09f/1
  State_psi_fd_SG_D_3_dfb80/1 -> Subtract_1c09f/2
  Subtract_eb416/1 -> Product_342c2/1
  Subtract_1c09f/1 -> Subtract_6df93/1
  Product_342c2/1 -> Subtract_6df93/2
  Subtract_6df93/1 -> Divide_c596a/1
  Constant_T_dd_28a4a/1 -> Divide_c596a/2
  Divide_c596a/1 -> Blockout_d_psi_fd_SG_D_3_68982/1
